simulink model "VSD_and_Park_transformation_6Phase"  (R2022a)
settings: Solver=FixedStepDiscrete  StartTime=0.0  StopTime=0.2  RelTol=1e-3
libraries: hdlsllib x4
settings Model: DataTypeOverride=Off  Creator=Andre Merx  LastModifiedBy=Andre Merx
settings SolverCC: AlgebraicLoopSolver=TrustRegion
settings DataIOCC: LimitDataPoints=on  SaveOutput=off  SaveTime=off
settings OptimizationCC: BlockReduction=off  ConditionallyExecuteInputs=off  DefaultParameterBehavior=Inlined  InheritOutputTypeSmallerThanSingle=on  LifeSpan=inf
settings DebuggingCC: AlgebraicLoopMsg=error  SingleTaskRateTransMsg=error  UnconnectedInputMsg=warning  UnconnectedOutputMsg=warning  UnconnectedLineMsg=warning  AllowSymbolicDim=off  StrictBusMsg=ErrorOnBusTreatedAsVector  SFUnexpectedBacktrackingDiag=warning  SFNoUnconditionalDefaultTransitionDiag=warning  SFExecutionAtInitializationDiag=none  SFMachineParentedDataDiag=warning  ArithmeticOperatorsInVariantConditions=warning
settings HardwareCC: ProdBitPerPointer=32  ProdBitPerSizeT=32  ProdBitPerPtrDiffT=32  ProdLargestAtomicFloat=None  ProdIntDivRoundTo=Undefined  ProdEndianess=Unspecified  ProdWordSize=32  ProdHWDeviceType=ASIC/FPGA->ASIC/FPGA  ProdEqTarget=off
settings SFSimCC: SimUseLocalCustomCode=off  CustomCodeUndefinedFunction=UseInterfaceOnly
settings RTWCC: RTWUseLocalCustomCode=off
settings CodeAppCC: StateflowObjectComments=on
settings GRTTargetCC: TargetLangStandard=C89/C90 (ANSI)
settings ConfigComp: CovScope=ReferencedModels  CovMetricSettings=dw  CovSaveCumulativeToWorkspaceVar=on  CovSaveSingleToWorkspaceVar=on  CovExternalEMLEnable=off  CovSFcnEnable=off

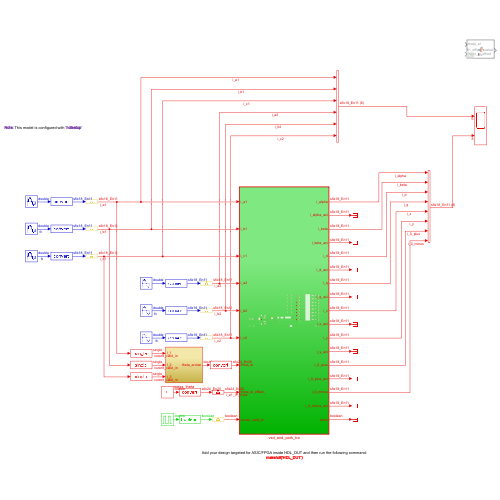
[thumbnail: Simulink's stored preview of the top-level diagram]
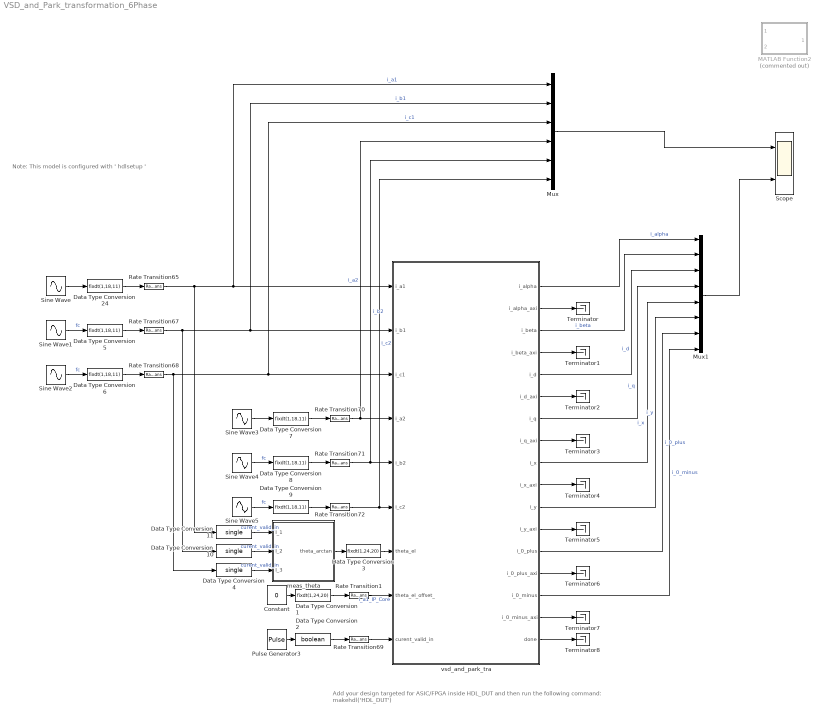
== system VSD_and_Park_transformation_6Phase ==
  note: Note: This model is configured with ' hdlsetup '
  note: Add your design targeted for ASIC/FPGA inside HDL_DUT and then run the following command:
      | makehdl('HDL_DUT')
  Constant : Constant  Value=0  SampleTime=-1
  Data Type Conversion1 : DataTypeConversion  OutDataTypeStr=fixdt(1,24,20)  SaturateOnIntegerOverflow=off  RndMeth=Floor
  Data Type Conversion10 : DataTypeConversion  OutDataTypeStr=single  SaturateOnIntegerOverflow=off  RndMeth=Floor
  Data Type Conversion11 : DataTypeConversion  OutDataTypeStr=single  SaturateOnIntegerOverflow=off  RndMeth=Floor
  Data Type Conversion2 : DataTypeConversion  OutDataTypeStr=boolean  SaturateOnIntegerOverflow=off  RndMeth=Floor
  Data Type Conversion{5..9,24} (6 alike) : DataTypeConversion  OutDataTypeStr=fixdt(1,18,11)  SaturateOnIntegerOverflow=off  RndMeth=Floor
  Data Type Conversion3 : DataTypeConversion  OutDataTypeStr=fixdt(1,24,20)  SaturateOnIntegerOverflow=off  RndMeth=Floor
  Data Type Conversion4 : DataTypeConversion  OutDataTypeStr=single  SaturateOnIntegerOverflow=off  RndMeth=Floor
  MATLAB Function2 : MATLAB Function  Commented=on  TreatAsAtomicUnit=on
  Mux : Mux  Inputs=6
  Mux1 : Mux  Inputs=8
  Pulse Generator3 : DiscretePulseGenerator  PulseType=Time based  Period=1/100000  PulseWidth=5
  Rate Transition{1,65,67..72} (8 alike) : RateTransition  OutPortSampleTime=1.0000e-08
  Scope : Scope  NumInputPorts=2
  Sine Wave : Sin  Frequency=100  SampleTime=1/100000
  Sine Wave1 : Sin  Frequency=100  Phase=(4/3)*pi  SampleTime=1/100000
  Sine Wave2 : Sin  Frequency=100  Phase=(2/3)*pi  SampleTime=1/100000
  Sine Wave3 : Sin  Amplitude=0.5  Frequency=100  Phase=-pi/6  SampleTime=1/100000
  Sine Wave4 : Sin  Amplitude=0.5  Frequency=100  Phase=(7/6)*pi  SampleTime=1/100000
  Sine Wave5 : Sin  Amplitude=0.5  Frequency=100  Phase=(1/2)*pi  SampleTime=1/100000
  Terminator{,1..8} (9 alike) : Terminator
  meas_theta : Subsystem
  vsd_and_park_tra : Subsystem  TreatAsAtomicUnit=on
  wires:
  Sine Wave/1 -> Data Type Conversion24/1
  Sine Wave1/1 -> Data Type Conversion5/1  "fc"
  Data Type Conversion6/1 -> Rate Transition68/1
  Sine Wave2/1 -> Data Type Conversion6/1  "fc"
  Data Type Conversion5/1 -> Rate Transition67/1
  Data Type Conversion24/1 -> Rate Transition65/1
  Rate Transition65/1 -> Mux/1, vsd_and_park_tra/1(i_a1), Data Type Conversion11/1  "i_a1"
  Rate Transition67/1 -> Mux/2, vsd_and_park_tra/2(i_b1), Data Type Conversion10/1  "i_b1"
  Rate Transition68/1 -> Mux/3, vsd_and_park_tra/3(i_c1), Data Type Conversion4/1  "i_c1"
  Sine Wave5/1 -> Data Type Conversion9/1  "fc"
  Data Type Conversion9/1 -> Rate Transition72/1
  Sine Wave4/1 -> Data Type Conversion8/1  "fc"
  Sine Wave3/1 -> Data Type Conversion7/1
  Data Type Conversion7/1 -> Rate Transition70/1
  Data Type Conversion8/1 -> Rate Transition71/1
  Rate Transition70/1 -> Mux/4, vsd_and_park_tra/4(i_a2)  "i_a2"
  Rate Transition71/1 -> Mux/5, vsd_and_park_tra/5(i_b2)  "i_b2"
  Rate Transition72/1 -> Mux/6, vsd_and_park_tra/6(i_c2)  "i_c2"
  meas_theta/1(theta_arctan) -> Data Type Conversion3/1
  Constant/1 -> Data Type Conversion1/1
  Data Type Conversion1/1 -> Rate Transition1/1
  Rate Transition1/1 -> vsd_and_park_tra/8(theta_el_offset_)  "i_a1_IP_Core"
  Pulse Generator3/1 -> Data Type Conversion2/1
  Rate Transition69/1 -> vsd_and_park_tra/9(curent_valid_in)
  Data Type Conversion2/1 -> Rate Transition69/1
  vsd_and_park_tra/2(i_alpha_axi) -> Terminator/1
  vsd_and_park_tra/4(i_beta_axi) -> Terminator1/1
  vsd_and_park_tra/6(i_d_axi) -> Terminator2/1
  vsd_and_park_tra/8(i_q_axi) -> Terminator3/1
  vsd_and_park_tra/10(i_x_axi) -> Terminator4/1
  vsd_and_park_tra/12(i_y_axi) -> Terminator5/1
  vsd_and_park_tra/14(i_0_plus_axi) -> Terminator6/1
  vsd_and_park_tra/16(i_0_minus_axi) -> Terminator7/1
  vsd_and_park_tra/17(done) -> Terminator8/1
  Mux/1 -> Scope/1
  vsd_and_park_tra/1(i_alpha) -> Mux1/1  "i_alpha"
  vsd_and_park_tra/3(i_beta) -> Mux1/2  "i_beta"
  vsd_and_park_tra/5(i_d) -> Mux1/3  "i_d"
  vsd_and_park_tra/7(i_q) -> Mux1/4  "i_q"
  vsd_and_park_tra/9(i_x) -> Mux1/5  "i_x"
  vsd_and_park_tra/11(i_y) -> Mux1/6  "i_y"
  vsd_and_park_tra/13(i_0_plus) -> Mux1/7  "i_0_plus"
  vsd_and_park_tra/15(i_0_minus) -> Mux1/8  "i_0_minus"
  Mux1/1 -> Scope/2
  Data Type Conversion3/1 -> vsd_and_park_tra/7(theta_el)
  Data Type Conversion4/1 -> meas_theta/3(I_3)  "curent_valid_in"
  Data Type Conversion10/1 -> meas_theta/2(I_2)  "curent_valid_in"
  Data Type Conversion11/1 -> meas_theta/1(I_1)  "curent_valid_in"

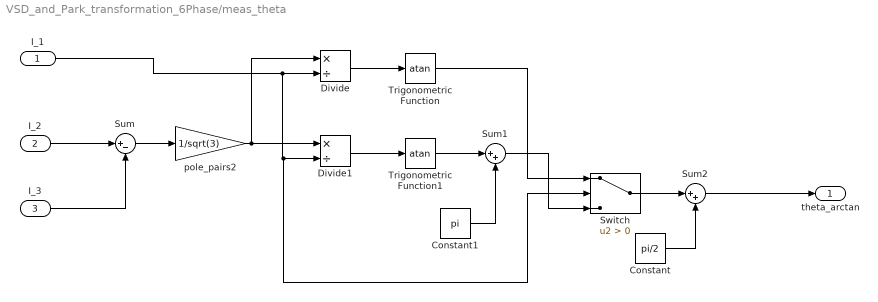
== system VSD_and_Park_transformation_6Phase/meas_theta ==
  I_1 : Inport
  I_2 : Inport  Port=2
  I_3 : Inport  Port=3
  Constant : Constant  Value=pi/2
  Constant1 : Constant  Value=pi
  Divide : Product  Inputs=*/
  Divide1 : Product  Inputs=*/
  Sum : Sum  Inputs=|+-
  Sum1 : Sum  Inputs=|++
  Sum2 : Sum  Inputs=|++
  Switch : Switch  Criteria=u2 > Threshold  SaturateOnIntegerOverflow=off  InputSameDT=off
  Trigonometric Function : Trigonometry  Operator=atan
  Trigonometric Function1 : Trigonometry  Operator=atan
  pole_pairs2 : Gain  Gain=1/sqrt(3)
  theta_arctan : Outport  VectorParamsAs1DForOutWhenUnconnected=off
  wires:
  Divide/1 -> Trigonometric Function/1
  Divide1/1 -> Trigonometric Function1/1
  Trigonometric Function1/1 -> Sum1/1
  pole_pairs2/1 -> Divide/1, Divide1/1
  Sum/1 -> pole_pairs2/1
  I_3/1 -> Sum/2
  I_2/1 -> Sum/1
  I_1/1 -> Switch/2, Divide1/2, Divide/2
  Sum1/1 -> Switch/3
  Trigonometric Function/1 -> Switch/1
  Switch/1 -> Sum2/1
  Constant/1 -> Sum2/2
  Constant1/1 -> Sum1/2
  Sum2/1 -> theta_arctan/1

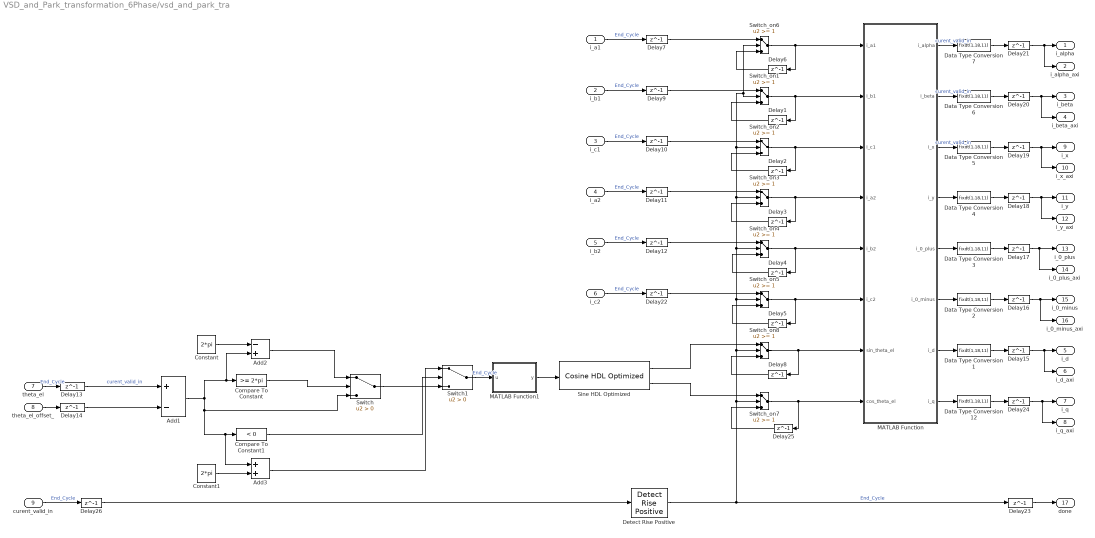
== system VSD_and_Park_transformation_6Phase/vsd_and_park_tra ==
  i_a1 : Inport
  i_b1 : Inport  Port=2
  i_c1 : Inport  Port=3
  i_a2 : Inport  Port=4
  i_b2 : Inport  Port=5
  i_c2 : Inport  Port=6
  theta_el : Inport  Port=7
  theta_el_offset_ : Inport  Port=8
  curent_valid_in : Inport  Port=9
  Add1 : Sum  Inputs=+-  OutDataTypeStr=Inherit: Same as accumulator  RndMeth=Simplest
  Add2 : Sum  Inputs=-+  RndMeth=Simplest
  Add3 : Sum  RndMeth=Simplest  OutDataTypeStr=Inherit: Same as first input
  Compare To Constant : hdlsllib/Logic and Bit Operations/Compare To Constant  relop=>=  const=2*pi  OutDataTypeStr=boolean
      settings: SourceProductBaseCode=SL
  Compare To Constant1 : hdlsllib/Logic and Bit Operations/Compare To Constant  relop=<  const=0  OutDataTypeStr=boolean
      settings: SourceProductBaseCode=SL
  Constant : Constant  Value=2*pi  OutDataTypeStr=fixdt(1,24,20)  SampleTime=1.0000e-08
  Constant1 : Constant  Value=2*pi  OutDataTypeStr=fixdt(1,24,20)  SampleTime=1.0000e-08
  Data Type Conversion{1..7,12} (8 alike) : DataTypeConversion  OutDataTypeStr=fixdt(1,18,11)  RndMeth=Simplest  SaturateOnIntegerOverflow=off
  Delay{1..26} (26 alike) : Delay  DelayLength=1
  Detect Rise Positive : hdlsllib/Logic and Bit Operations/Detect Rise Positive  vinit=0  OutDataTypeStr=boolean
      settings: SourceProductBaseCode=SL
  MATLAB Function : MATLAB Function  TreatAsAtomicUnit=on
  MATLAB Function1 : MATLAB Function  TreatAsAtomicUnit=on
  Sine HDL Optimized : hdlsllib/Lookup Tables/Cosine HDL Optimized  OutputFormula=sin(2*pi*u) and cos(2*pi*u)  NumDataPoints=512  TableDataTypeStr=fixdt(1,17,11)  SimulateLUTROMDelay=off
      settings: SourceProductBaseCode=SL
  Switch : Switch  Criteria=u2 > Threshold  OutDataTypeStr=fixdt(1,24,20)  RndMeth=Simplest  SaturateOnIntegerOverflow=off  InputSameDT=off
  Switch1 : Switch  Criteria=u2 > Threshold  OutDataTypeStr=fixdt(1,24,20)  RndMeth=Simplest  SaturateOnIntegerOverflow=off  InputSameDT=off
  Switch_on{1..8} (8 alike) : Switch  Threshold=1  RndMeth=Simplest  SaturateOnIntegerOverflow=off  InputSameDT=off  OutDataTypeStr=Inherit: Same as first input
  i_alpha : Outport
  i_alpha_axi : Outport  Port=2
  i_beta : Outport  Port=3
  i_beta_axi : Outport  Port=4
  i_d : Outport  Port=5
  i_d_axi : Outport  Port=6
  i_q : Outport  Port=7
  i_q_axi : Outport  Port=8
  i_x : Outport  Port=9
  i_x_axi : Outport  Port=10
  i_y : Outport  Port=11
  i_y_axi : Outport  Port=12
  i_0_plus : Outport  Port=13
  i_0_plus_axi : Outport  Port=14
  i_0_minus : Outport  Port=15
  i_0_minus_axi : Outport  Port=16
  done : Outport  Port=17
  wires:
  theta_el_offset_/1 -> Delay14/1
  i_c2/1 -> Delay22/1  "End_Cycle"
  Switch_on8/1 -> Delay8/1, MATLAB Function/7(sin_theta_el)
  Delay8/1 -> Switch_on8/3
  Detect Rise Positive/1 -> Delay23/1, Switch_on7/2, Switch_on6/2, Switch_on1/2, Switch_on2/2, Switch_on3/2, Switch_on4/2, Switch_on5/2, Switch_on8/2  "End_Cycle"
  Delay4/1 -> Switch_on4/3
  Switch_on2/1 -> Delay2/1, MATLAB Function/3(i_c1)
  Delay1/1 -> Switch_on1/3
  Switch_on1/1 -> Delay1/1, MATLAB Function/2(i_b1)
  Switch_on6/1 -> MATLAB Function/1(i_a1), Delay6/1
  Switch_on4/1 -> Delay4/1, MATLAB Function/5(i_b2)
  curent_valid_in/1 -> Delay26/1  "End_Cycle"
  Switch/1 -> Switch1/3
  Switch_on3/1 -> MATLAB Function/4(i_a2), Delay3/1
  Delay6/1 -> Switch_on6/3
  Constant/1 -> Add2/1
  Add1/1 -> Switch/3, Compare To Constant1/1, Add3/1, Compare To Constant/1, Add2/2
  Delay2/1 -> Switch_on2/3
  Constant1/1 -> Add3/2
  theta_el/1 -> Delay13/1  "End_Cycle"
  Delay3/1 -> Switch_on3/3
  i_a1/1 -> Delay7/1  "End_Cycle"
  i_b2/1 -> Delay12/1  "End_Cycle"
  Add2/1 -> Switch/1
  i_a2/1 -> Delay11/1  "End_Cycle"
  i_b1/1 -> Delay9/1  "End_Cycle"
  Delay5/1 -> Switch_on5/3
  Add3/1 -> Switch1/1
  i_c1/1 -> Delay10/1  "End_Cycle"
  Switch_on5/1 -> Delay5/1, MATLAB Function/6(i_c2)
  MATLAB Function/4(i_y) -> Data Type Conversion4/1
  MATLAB Function/5(i_0_plus) -> Data Type Conversion3/1
  MATLAB Function/6(i_0_minus) -> Data Type Conversion2/1
  MATLAB Function/7(i_d) -> Data Type Conversion1/1
  MATLAB Function/8(i_q) -> Data Type Conversion12/1
  Delay23/1 -> done/1
  MATLAB Function/1(i_alpha) -> Data Type Conversion7/1  "curent_valid_in"
  MATLAB Function/2(i_beta) -> Data Type Conversion6/1  "curent_valid_in"
  MATLAB Function/3(i_x) -> Data Type Conversion5/1  "curent_valid_in"
  Delay24/1 -> i_q_axi/1, i_q/1
  Delay15/1 -> i_d_axi/1, i_d/1
  Delay16/1 -> i_0_minus_axi/1, i_0_minus/1
  Delay17/1 -> i_0_plus_axi/1, i_0_plus/1
  Delay18/1 -> i_y_axi/1, i_y/1
  Delay19/1 -> i_x_axi/1, i_x/1
  Delay20/1 -> i_beta_axi/1, i_beta/1
  Delay21/1 -> i_alpha_axi/1, i_alpha/1
  Delay7/1 -> Switch_on6/1
  Delay9/1 -> Switch_on1/1
  Delay10/1 -> Switch_on2/1
  Delay11/1 -> Switch_on3/1
  Delay12/1 -> Switch_on4/1
  Delay22/1 -> Switch_on5/1
  Delay26/1 -> Detect Rise Positive/1
  Data Type Conversion12/1 -> Delay24/1
  Data Type Conversion1/1 -> Delay15/1
  Data Type Conversion2/1 -> Delay16/1
  Data Type Conversion3/1 -> Delay17/1
  Data Type Conversion4/1 -> Delay18/1
  Data Type Conversion5/1 -> Delay19/1
  Data Type Conversion6/1 -> Delay20/1
  Data Type Conversion7/1 -> Delay21/1
  Compare To Constant/1 -> Switch/2
  Compare To Constant1/1 -> Switch1/2
  Switch_on7/1 -> Delay25/1, MATLAB Function/8(cos_theta_el)
  Delay25/1 -> Switch_on7/3
  Sine HDL Optimized/1 -> Switch_on8/1
  Sine HDL Optimized/2 -> Switch_on7/1
  Delay13/1 -> Add1/1  "curent_valid_in"
  Delay14/1 -> Add1/2
  Switch1/1 -> MATLAB Function1/1(u)  "End_Cycle"
  MATLAB Function1/1(y) -> Sine HDL Optimized/1

== matlab function VSD_and_Park_transformation_6Phase/vsd_and_park_tra/MATLAB Function1 ==
  settings: fimath=fimath('RoundingMethod', 'Floor','OverflowAction', 'Wrap','ProductMode', 'FullPrecision', 'SumMode', 'FullPrecision')
  data: u input; y output
function y = fcn(u)

    y = u*(1/(2*pi));

end

== matlab function VSD_and_Park_transformation_6Phase/vsd_and_park_tra/MATLAB Function ==
  settings: fimath=fimath('RoundingMethod', 'Floor','OverflowAction', 'Wrap','ProductMode', 'FullPrecision', 'SumMode', 'FullPrecision')
  data: i_a1 input; i_alpha output; i_b1 input; i_c1 input; i_a2 input; i_b2 input; i_c2 input; sin_theta_el input; i_beta output; i_x output; i_y output; i_0_plus output; i_0_minus output; i_d output; i_q output; cos_theta_el input
function [i_alpha,i_beta,i_x,i_y,i_0_plus,i_0_minus,i_d,i_q] = VSD_and_Park_transformation(i_a1,i_b1,i_c1,i_a2,i_b2,i_c2,sin_theta_el,cos_theta_el)

    % VSD-Transformation
    A = [0 0 0 0 0 0]';

    A =  0.3333*[1    -0.5        -0.5        0.8660   -0.8660  0 ;
                0    0.8660   -0.8660  0.5         0.5         -1;
                1    -0.5        -0.5        -0.8660  0.8660   0 ;
                0    -0.8660  0.8660   0.5         0.5         -1;
                1    1           1           0           0           0 ;
                0    0           0           1           1           1] * [i_a1 i_b1 i_c1 i_a2 i_b2 i_c2]';

    i_alpha = A(1);
    i_beta = A(2);
    i_x = A(3);
    i_y = A(4);
    i_0_plus = A(5);
    i_0_minus = A(6);

    % Park-Transformation
%    B = [0 0]';

%     B = [cos(theta_el)       sin(theta_el);
%         -sin(theta_el)       cos(theta_el)] * [i_alpha i_beta]';

 %   i_d = B(1);
 %   i_q = B(2);



i_d = cos_theta_el*i_alpha+sin_theta_el*i_beta;
i_q = -sin_theta_el*i_alpha+cos_theta_el*i_beta;


end

== matlab function VSD_and_Park_transformation_6Phase/MATLAB Function2 ==
  data: theta_el input; theta_el_with_offset_scaled output; theta_el_offset input
function theta_el_with_offset_scaled = fcn(theta_el, theta_el_offset)

theta_el_with_offset = theta_el-theta_el_offset;


if theta_el_with_offset>=(2*pi)
    theta_el_with_offset_scaled = theta_el_with_offset-2*pi;
else
    theta_el_with_offset_scaled = theta_el_with_offset+0;
end

if theta_el_with_offset<(2*pi)
    theta_el_with_offset_scaled = theta_el_with_offset+2*pi;
end

end
